simulink library "vmc"  (R2021b)
settings: Solver=VariableStepAuto  StartTime=0.0  StopTime=10.0  RelTol=1e-3
undefined symbols (not defined in the file or in its folder): AVMC_ACCDeltaTqIGain_X_kph, AVMC_ACCDeltaTqIGain_Y_mps2, AVMC_ACCDeltaTqPGain_X_kph, AVMC_ACCDeltaTqPGain_Y_kph, AVMC_ACCLongSteadyCtrl_X_kph, AVMC_AggressJerkPCT4AT_X_kph, AVMC_AggressJerkPCT_X_kph, AVMC_AggressLimitPCT4AT_X_kph, AVMC_AggressLimitPCT_X_kph, AVMC_CCLongSteadyCtrl_X_kph, AVMC_DISCDeltaTqIGain_X_kph, AVMC_DISCDeltaTqIGain_Y_mps2, AVMC_DISCDeltaTqPGain_X_kph, AVMC_DISCDeltaTqPGain_Y_kph, AVMC_DISCTrunAccJerk_X_s, AVMC_DISCTrunAccLimit_X_s, AVMC_ESCRegenOut_X_kph, AVMC_ESCRegenOut_Y_Deg, AVMC_ESCRegenOutEnSpd_X_Deg, AVMC_ISOAccLimit_X_mps, AVMC_ISODecLimit_X_mps, AVMC_ISOJerk_X_mps, AVMC_LatESCRegenOut_X_kph, AVMC_LatESCRegenOut_Y_Deg, AVMC_LongAccDeadZone_X_kph, AVMC_LongAccFiltTsforP2_X_Gps, AVMC_MCPresBaseTq_X_bar, AVMC_MSALongSteadyCtrl_X_kph, AVMC_MSAPedalOvrd2_X_kph, AVMC_MSAPedalOvrd_X_kph, AVMC_MSASpdBand_X_kph, AVMC_MSATqDownEndTq_X_kph, AVMC_MSATqDownTime_X_kph, AVMC_OPDDisSlideRate_X_Deg, AVMC_RDCDetectTime_X_kph, AVMC_RDCDetectTime_Y_pct, AVMC_RDCEnSlideRate_X_Deg, AVMC_RearWhlTqRatio_X_Nm, AVMC_RearWhlTqRatio_Y_gps, AVMC_RearWhlTqSlipGain_X_rat, AVMC_RearWhlTqSlipGain_Y_kph, AVMC_RearWhlTqSTRGGain_X_deg, AVMC_RearWhlTqSTRGGain_Y_kph, AVMC_RWSRrTSA2RWSPos_X_deg, AVMC_RWSSAS2FrtTSA_X_deg, AVMC_RWSVehSPD2RWSCoef_X_kph, AVMC_SoftJerkPCT_X_kph, AVMC_SoftLimitPCT_X_kph, AVMC_StESCYaw_X_kph, AVMC_StESCYaw_Y_Deg, AVMC_StESCYawCom_X_kph, AVMC_StESCYawCom_Y_Gps, AVMC_TMSpdBaseTq_X_rpm, AVMC_VehHoldBDecMap_X_kph, AVMC_VehHoldDecCtrlTime_X_kph, AVMC_VehHoldMCPPass_X_deg, C_TASK_10MS_S, C_TASK_5MS_S, DEG2RAD, ENUM_ACCAVAIL_AVAILABLE ... (+409)
libraries: hcu_lib x74, simulink x68, simulink_extras x3, $bdroot x2
(part 8 of 15)

== system vmc/VMC/VMC/CruiseControlFunction/CCDemandTorqueCalculation ==
  VVMC_FeatSetSpdForCalcu_kph : Inport
  VINP_VehSpeed_kph : Inport  Port=2
  VVMC_CruzActive_flg : Inport  Port=3
  VTQD_DriverWhlTqDem_Nm : Inport  Port=4
  VVMC_LongAcc_Gps : Inport  Port=5
  VVMC_CCPedalOvrd_flg : Inport  Port=6
  VVMC_CalMeterSpeed_kph : Inport  Port=7
  VVMC_FeatArbitrFinal_enum : Inport  Port=8
  VVMC_ActACCRequiredAccel_mps2 : Inport  Port=9
  VVMC_MeterIndSpeedForCalcu_kph : Inport  Port=10
  VVMC_SafetyCtrl_flg : Inport  Port=11
  VTQR_FrTMTqReq_Nm : Inport  Port=12
  VTQR_RrTMTqReq_Nm : Inport  Port=13
  VVMC_TotalAvailBrkRgnTq_Nm : Inport  Port=14
  AND12 : Logic  AllPortsSameDT=off  OutDataTypeStr=boolean
  Abs3 : Abs
  Abs4 : Abs
  Add{8,12,16,20..21} (5 alike) : Sum
  Add22 : Sum  Inputs=+-
  Add23 : Sum  Inputs=+-
  Cast To Single4 : DataTypeConversion  OutDataTypeStr=single
  Cast To Single5 : DataTypeConversion  OutDataTypeStr=single
  Constant1 : Constant  Value=KVMC_CCTqUpLim_Nm
  Constant104 : Constant  Value=ZERO_FLOAT
  Constant105 : Constant  Value=KTQD_RrTMTotalGearRatio_gain
  Constant106 : Constant  Value=KTQR_RrTMGearEff_c
  Constant107 : Constant  Value=KVMC_GravityValue_mps2
  Constant2 : Constant  Value=KVMC_CCTqLowLim_Nm
  Constant3 : Constant  Value=ZERO_FLOAT
  Constant36 : Constant  Value=KVMC_AccDevLowLim_mps2
  Constant38 : Constant  Value=KVMC_AccDevUpLim_mps2
  Constant4 : Constant  Value=KVMC_CCDISCPGainSW_flg
  Constant40 : Constant  Value=KVMC_CCSpdDevUpLim_kph
  Constant5 : Constant  Value=KVMC_CCTqUpLim_Nm
  Constant56 : Constant  Value=KVMC_CCSpdDevLowLim_kph
  Constant58 : Constant  Value=KVMC_Veh2MeterSpdFactor_enum
  Constant59 : Constant  Value=KVMC_Veh2MeterSpdOffset_enum
  Constant6 : Constant  Value=KVMC_CCTqLowLim_Nm
  Constant64 : Constant  Value=KVMC_TqSafetyCtrl_flg
  Constant65 : Constant  Value=KVMC_Veh2MeterSpdLoFactor_enum
  Constant7 : Constant  Value=ZERO_FLOAT
  Constant71 : Constant  Value=KTQR_FrTMGearEff_c
  Constant76 : Constant  Value=KTQD_FrTMTotalGearRatio_gain
  Data Type Conversion1 : DataTypeConversion  OutDataTypeStr=single
  Detect Decrease3 : simulink/Logic and Bit Operations/Detect Decrease  vinit=0.0  OutDataTypeStr=boolean
  Detect Increase3 : simulink/Logic and Bit Operations/Detect Increase  vinit=0.0  OutDataTypeStr=boolean
  Divide11 : Product  Inputs=**
  Divide12 : Product  Inputs=**
  Divide4 : Product  Inputs=***
  Divide7 : Product  Inputs=***
  InitialCondition: 1 : UnitDelay  SampleTime=-1  HasFrameUpgradeWarning=on
  Logical Operator1 : Logic  Operator=OR  AllPortsSameDT=off  OutDataTypeStr=boolean
  MVMC_DISCDeltaTqIGain_Z_Nm : Lookup_n-D  BreakpointsForDimension1=AVMC_DISCDeltaTqIGain_Y_mps2  BreakpointsForDimension2=AVMC_DISCDeltaTqIGain_X_kph  Table=MVMC_DISCDeltaTqIGain_Z_Nm  InternalRulePriority=Speed  RndMeth=Simplest  InputSameDT=on
      settings: InputPortMap=u0,u1
  MVMC_DISCDeltaTqPGain_Z_Nm : Lookup_n-D  BreakpointsForDimension1=AVMC_DISCDeltaTqPGain_Y_kph  BreakpointsForDimension2=AVMC_DISCDeltaTqPGain_X_kph  BreakpointsForDimension3=[5, 7]  Table=MVMC_DISCDeltaTqPGain_Z_Nm  ExtrapMethod=Clip  InternalRulePriority=Speed  RndMeth=Simplest  InputSameDT=on
      settings: InputPortMap=u0,u1
  Max : MinMax  Function=max  Inputs=2
  Max1 : MinMax  Function=max  Inputs=2
  Product2 : Product
  Relational Operator18 : RelationalOperator  Operator=<=  OutDataTypeStr=boolean  RndMeth=Simplest
  Saturation Dynamic{1,7..9} (4 alike) : simulink/Discontinuities/Saturation Dynamic  OutMin=[]  OutMax=[]  OutDataTypeStr=Inherit: Same as second input  OutDataType=fixdt(1, 16)  OutScaling=2^-10  DoSatur=off
  Switch{,2,5,7} (4 alike) : Switch  Criteria=u2 > Threshold
  Switch1 : Switch  Criteria=u2 > Threshold  Threshold=KVMC_Veh2MeterSpdLoBdy_kph
  Unit Delay3 : UnitDelay  SampleTime=-1  HasFrameUpgradeWarning=on
  u2 > 0 (3)1 : Switch  Criteria=u2 > Threshold
  u2 > 0 (4)1 : Switch  Criteria=u2 > Threshold
  VVMC_CruzWhlTqCal_Nm : Outport
  wires:
  VVMC_FeatSetSpdForCalcu_kph/1 -> [VVMC_FeatSetSpdForCalcu_kph]
  VTQD_DriverWhlTqDem_Nm/1 -> [VTQD_DriverWhlTqDem_Nm]
  VVMC_CruzActive_flg/1 -> [VVMC_CruzActive_flg]
  VINP_VehSpeed_kph/1 -> [VINP_VehSpeed_kph]
  [VVMC_CruzWhlTqCal_Nm] -> VVMC_CruzWhlTqCal_Nm/1
  VVMC_LongAcc_Gps/1 -> [VVMC_LongAcc_Gps]
  VVMC_CCPedalOvrd_flg/1 -> [VVMC_CCPedalOvrd_flg]
  VVMC_CalMeterSpeed_kph/1 -> [VVMC_CalMeterSpeed_kph]
  VVMC_FeatArbitrFinal_enum/1 -> [VVMC_FeatArbitrFinal_enum]
  VVMC_ActACCRequiredAccel_mps2/1 -> [VVMC_CCReqAcc_mps2]
  VVMC_MeterIndSpeedForCalcu_kph/1 -> [VVMC_MeterIndSpeedForCalcu_kph]
  VVMC_SafetyCtrl_flg/1 -> [VVMC_SafetyCtrl_flg]
  Switch5/1 -> Cast To Single5/1
  Detect Decrease3/1 -> Logical Operator1/2
  Divide4/1 -> Add16/1
  [VVMC_CruzActive_flg] -> Detect Increase3/1
  [VVMC_FeatSetSpdForCalcu_kph] -> MVMC_DISCDeltaTqPGain_Z_Nm/2
  Data Type Conversion1/1 -> Add23/1
  u2 > 0 (3)1/1 -> Switch5/1
  Constant71/1 -> Divide4/3
  Constant106/1 -> Divide7/3
  [VVMC_SafetyCtrl_flg] -> AND12/2
  Saturation Dynamic9/1 -> MVMC_DISCDeltaTqPGain_Z_Nm/1
  Relational Operator18/1 -> u2 > 0 (4)1/2
  [VVMC_LastCCWhlTqCalW_Nm] -> Abs3/1, u2 > 0 (4)1/1
  u2 > 0 (4)1/1 -> u2 > 0 (3)1/1
  [VTQR_RrTMTqReq_Nm] -> Divide7/1
  [VVMC_LastCCWhlTqCalW_Nm] -> Add12/1
  MVMC_DISCDeltaTqIGain_Z_Nm/1 -> [VVMC_CCIGainDeltaTq_Nm]
  Add23/1 -> Saturation Dynamic9/2
  Constant104/1 -> Switch5/3
  InitialCondition: 1/1 -> [VVMC_LastCCWhlTqCalW_Nm]  "VVMC_LastCruzWhlTqCal_Nm"
  Detect Increase3/1 -> Logical Operator1/1
  [VINP_VehSpeed_kph] -> MVMC_DISCDeltaTqIGain_Z_Nm/2
  [VVMC_CCIGainDeltaTq_Nm] -> Add12/2
  Abs4/1 -> Relational Operator18/2
  Saturation Dynamic7/1 -> InitialCondition: 1/1, Add21/2
  Abs3/1 -> Relational Operator18/1
  [VTQR_FrTMTqReq_Nm] -> Divide4/1
  Saturation Dynamic8/1 -> MVMC_DISCDeltaTqIGain_Z_Nm/1
  [VVMC_CCIGainDeltaTq_Nm] -> Add20/2
  Constant76/1 -> Divide4/2
  Divide7/1 -> Add16/2
  AND12/1 -> u2 > 0 (3)1/2
  Add20/1 -> Switch7/1
  Constant105/1 -> Divide7/2
  [VVMC_CruzActive_flg] -> Switch5/2
  [VVMC_CCPedalOvrd_flg] -> Unit Delay3/1
  Cast To Single5/1 -> Saturation Dynamic7/2
  Switch7/1 -> Cast To Single4/1
  Add12/1 -> Switch7/3
  Constant40/1 -> Saturation Dynamic9/1
  Constant5/1 -> Saturation Dynamic7/1
  Add16/1 -> Add20/1
  Unit Delay3/1 -> Detect Decrease3/1
  [VVMC_CCReqAcc_mps2] -> Add22/1
  Add22/1 -> Saturation Dynamic8/2
  Constant107/1 -> Product2/2
  Constant64/1 -> AND12/1
  [VVMC_FeatSetSpdForCalcu_kph] -> Data Type Conversion1/1
  Logical Operator1/1 -> Switch7/2
  Constant38/1 -> Saturation Dynamic8/1
  Product2/1 -> Add22/2
  [VVMC_LongAcc_Gps] -> Product2/1
  Constant36/1 -> Saturation Dynamic8/3
  Constant6/1 -> Max/1
  Constant56/1 -> Saturation Dynamic9/3
  Cast To Single4/1 -> u2 > 0 (4)1/3, Abs4/1, u2 > 0 (3)1/3
  VTQR_FrTMTqReq_Nm/1 -> [VTQR_FrTMTqReq_Nm]
  VTQR_RrTMTqReq_Nm/1 -> [VTQR_RrTMTqReq_Nm]
  VVMC_TotalAvailBrkRgnTq_Nm/1 -> [VVMC_TotalAvailBrkRgnTq_Nm]
  [VVMC_TotalAvailBrkRgnTq_Nm] -> Max/2
  Max/1 -> Saturation Dynamic7/3
  Switch/1 -> [VVMC_CCPGainDeltaTq_Nm]
  Switch2/1 -> Add21/1
  [VVMC_CCPGainDeltaTq_Nm] -> Switch2/1
  Constant4/1 -> Switch2/2
  Constant7/1 -> Switch2/3
  Saturation Dynamic1/1 -> [VVMC_CruzWhlTqCal_Nm]  "VVMC_CruzWhlTqCal_Nm"
  [VINP_VehSpeed_kph] -> Divide11/2, Switch1/2, Divide12/1
  Switch1/1 -> Add23/2
  Constant59/1 -> Add8/1
  Add8/1 -> Switch1/1
  Constant58/1 -> Divide11/1
  Constant65/1 -> Divide12/2
  Divide11/1 -> Add8/2
  Divide12/1 -> Switch1/3
  Max1/1 -> Saturation Dynamic1/3
  [VVMC_TotalAvailBrkRgnTq_Nm] -> Max1/2
  Constant2/1 -> Max1/1
  Constant1/1 -> Saturation Dynamic1/1
  Add21/1 -> Saturation Dynamic1/2
  [VVMC_CruzActive_flg] -> Switch/2
  MVMC_DISCDeltaTqPGain_Z_Nm/1 -> Switch/1
  Constant3/1 -> Switch/3

== system vmc/VMC/VMC/CruiseControlFunction/CCTorqueSourceDetermination ==
  VTQD_DriverWhlTqDem_Nm : Inport
  VVMC_CruzWhlTqCal_Nm : Inport  Port=2
  VTQD_LowIdleAccPedal_flg : Inport  Port=3
  VTQD_RegenMode_enum : Inport  Port=4
  VVMC_FeatArbitrFinal_enum : Inport  Port=5
  task_time_s : Inport  Port=6
  AND1 : Logic  Inputs=3  AllPortsSameDT=off  OutDataTypeStr=boolean
  Add : Sum
  Constant20 : Constant  Value=FALSE
  Constant21 : Constant  Value=ENUM_FEATARBITRSTA_CC
  Constant22 : Constant  Value=TRUE
  Constant23 : Constant  Value=KVMC_ACCPedalOvrdRestTime_s
  DelayEnable : hcu_lib/Basic_Blocks/DelayEnable
  Direct Lookup Table (n-D)1 : LookupNDDirect  NumberOfTableDimensions=1  Table=MVMC_ACCPedalOvrdTqHys_Y_Nm
  NOT2 : Logic  Operator=NOT  AllPortsSameDT=off  OutDataTypeStr=boolean
  OR1 : Logic  Operator=OR  AllPortsSameDT=off  OutDataTypeStr=boolean
  Relational Operator6 : RelationalOperator  Operator===  OutDataTypeStr=boolean  RndMeth=Simplest
  Relational Operator7 : RelationalOperator  Operator=>  OutDataTypeStr=boolean  RndMeth=Simplest
  Relational Operator8 : RelationalOperator  Operator=<=  OutDataTypeStr=boolean  RndMeth=Simplest
  SR_Latch : hcu_lib/Basic_Blocks/SR_Latch
  u2 > 0 (1) : Switch  Criteria=u2 > Threshold
  u2 > 0 (2) : Switch  Criteria=u2 > Threshold
  VVMC_CruzWhlTqReq_Nm : Outport
  VVMC_CCPedalOvrd_flg : Outport  Port=2
  wires:
  VTQD_DriverWhlTqDem_Nm/1 -> [VTQD_DriverWhlTqDem_Nm]
  VVMC_CruzWhlTqCal_Nm/1 -> [VVMC_CruzWhlTqCal_Nm]
  [VVMC_CruzWhlTqReq_Nm] -> VVMC_CruzWhlTqReq_Nm/1
  VTQD_LowIdleAccPedal_flg/1 -> [VTQD_LowIdleAccPedal_flg]
  [VVMC_CCPedalOvrd_flg] -> VVMC_CCPedalOvrd_flg/1
  [task_time_s] -> DelayEnable/3
  [VTQD_LowIdleAccPedal_flg] -> NOT2/1
  [VTQD_DriverWhlTqDem_Nm] -> u2 > 0 (1)/1
  [VVMC_CruzWhlTqCal_Nm] -> u2 > 0 (1)/3
  [VVMC_CruzWhlTqCal_Nm] -> Relational Operator8/2
  [VVMC_CruzWhlTqCal_Nm] -> Add/1
  u2 > 0 (2)/1 -> [VVMC_CCPedalOvrd_flg]
  Add/1 -> Relational Operator7/2
  [VTQD_DriverWhlTqDem_Nm] -> Relational Operator7/1
  [VVMC_FeatArbitrFinal_enum] -> Relational Operator6/1
  OR1/1 -> SR_Latch/2
  Relational Operator8/1 -> DelayEnable/1
  Constant23/1 -> DelayEnable/2
  u2 > 0 (1)/1 -> [VVMC_CruzWhlTqReq_Nm]
  Relational Operator7/1 -> SR_Latch/1
  [VVMC_CCPedalTqEnOvrd_flg] -> AND1/3
  NOT2/1 -> AND1/2
  Constant20/1 -> u2 > 0 (2)/3
  Relational Operator6/1 -> AND1/1
  [VTQD_RegenMode_enum] -> Direct Lookup Table (n-D)1/1
  [VTQD_DriverWhlTqDem_Nm] -> Relational Operator8/1
  DelayEnable/1 -> OR1/1
  SR_Latch/1 -> [VVMC_CCPedalTqEnOvrd_flg]
  [VTQD_LowIdleAccPedal_flg] -> OR1/2
  AND1/1 -> u2 > 0 (1)/2, u2 > 0 (2)/2
  Constant21/1 -> Relational Operator6/2
  Direct Lookup Table (n-D)1/1 -> Add/2
  Constant22/1 -> u2 > 0 (2)/1
  VTQD_RegenMode_enum/1 -> [VTQD_RegenMode_enum]
  VVMC_FeatArbitrFinal_enum/1 -> [VVMC_FeatArbitrFinal_enum]
  task_time_s/1 -> [task_time_s]

== system vmc/VMC/VMC/IMU/IMU memorized offset result ==
  VINP_MemOffsetGyroX_raw16 : Inport
  VINP_MemOffsetGyroY_raw16 : Inport  Port=2
  VINP_MemOffsetGyroZ_raw16 : Inport  Port=3
  VINP_MemOffsetAccX_raw16 : Inport  Port=4
  VINP_MemOffsetAccY_raw16 : Inport  Port=5
  VINP_MemOffsetAccZ_raw16 : Inport  Port=6
  ACCEL_FS_SEL = 001 SENSITIVITY = 2000 LSB/g : Constant  Value=2000
  Constant6 : Constant  Value=ONE_FLOAT  OutDataTypeStr=single
  Data Type Conversion : DataTypeConversion  OutDataTypeStr=uint16
  Data Type Conversion{1..6} (6 alike) : DataTypeConversion  OutDataTypeStr=single
  Data Type Conversion7 : DataTypeConversion  OutDataTypeStr=uint16
  Divide{,1..5} (6 alike) : Product  Inputs=**
  GYRO_FS_SEL = 0001 SENSITIVITY = 50 LSB/dps : Constant  Value=50
  Math Function{,1..5} (6 alike) : Math  Operator=reciprocal  SaturateOnIntegerOverflow=on
  Plus : Sum  Inputs=+-
  VVMC_MemOffsetGyroX_Dps : Outport
  VVMC_MemOffsetGyroY_Dps : Outport  Port=2
  VVMC_MemOffsetGyroZ_Dps : Outport  Port=3
  VVMC_MemOffsetAccX_G : Outport  Port=4
  VVMC_MemOffsetAccY_G : Outport  Port=5
  VVMC_MemOffsetAccZ_G : Outport  Port=6
  wires:
  VINP_MemOffsetGyroX_raw16/1 -> [VINP_MemOffsetGyroX_raw16]
  VINP_MemOffsetGyroY_raw16/1 -> [VINP_MemOffsetGyroY_raw16]
  [VINP_MemOffsetGyroX_raw16] -> Divide/1
  [VVMC_GyroFSCalSet_enum] -> Data Type Conversion1/1
  GYRO_FS_SEL = 0001 SENSITIVITY = 50 LSB/dps/1 -> Data Type Conversion/1
  Data Type Conversion/1 -> [VVMC_GyroFSCalSet_enum]  "VVMC_GyroFSCalSet_enum"
  [VVMC_GyroFSCalSet_enum] -> Data Type Conversion2/1
  [VINP_MemOffsetGyroY_raw16] -> Divide1/1
  [VINP_MemOffsetGyroZ_raw16] -> Divide2/1
  [VVMC_GyroFSCalSet_enum] -> Data Type Conversion3/1
  [VVMC_AccFSCalSet_enum] -> Data Type Conversion4/1
  [VINP_MemOffsetAccX_raw16] -> Divide3/1
  [VINP_MemOffsetAccY_raw16] -> Divide4/1
  [VVMC_AccFSCalSet_enum] -> Data Type Conversion5/1
  [VVMC_AccFSCalSet_enum] -> Data Type Conversion6/1
  [VINP_MemOffsetAccZ_raw16] -> Divide5/1
  Data Type Conversion7/1 -> [VVMC_AccFSCalSet_enum]  "VVMC_AccFSCalSet_enum"
  ACCEL_FS_SEL = 001 SENSITIVITY = 2000 LSB/g/1 -> Data Type Conversion7/1
  Divide/1 -> [VVMC_MemOffsetGyroX_Dps]  "VVMC_MemOffsetGyroX_Dps"
  Divide1/1 -> [VVMC_MemOffsetGyroY_Dps]  "VVMC_MemOffsetGyroY_Dps"
  Divide2/1 -> [VVMC_MemOffsetGyroZ_Dps]  "VVMC_MemOffsetGyroZ_Dps"
  Divide3/1 -> [VVMC_MemOffsetAccX_G]  "VVMC_MemOffsetAccX_G"
  Plus/1 -> [VVMC_MemOffsetAccZ_G]  "VVMC_MemOffsetAccZ_G"
  Divide5/1 -> Plus/1
  Constant6/1 -> Plus/2
  [VVMC_MemOffsetGyroX_Dps] -> VVMC_MemOffsetGyroX_Dps/1
  [VVMC_MemOffsetGyroY_Dps] -> VVMC_MemOffsetGyroY_Dps/1
  [VVMC_MemOffsetGyroZ_Dps] -> VVMC_MemOffsetGyroZ_Dps/1
  [VVMC_MemOffsetAccX_G] -> VVMC_MemOffsetAccX_G/1
  [VVMC_MemOffsetAccY_G] -> VVMC_MemOffsetAccY_G/1
  [VVMC_MemOffsetAccZ_G] -> VVMC_MemOffsetAccZ_G/1
  Divide4/1 -> [VVMC_MemOffsetAccY_G]  "VVMC_MemOffsetAccY_G"
  VINP_MemOffsetGyroZ_raw16/1 -> [VINP_MemOffsetGyroZ_raw16]
  VINP_MemOffsetAccX_raw16/1 -> [VINP_MemOffsetAccX_raw16]
  VINP_MemOffsetAccY_raw16/1 -> [VINP_MemOffsetAccY_raw16]
  VINP_MemOffsetAccZ_raw16/1 -> [VINP_MemOffsetAccZ_raw16]
  Math Function/1 -> Divide/2
  Math Function1/1 -> Divide1/2
  Math Function2/1 -> Divide2/2
  Math Function3/1 -> Divide3/2
  Math Function4/1 -> Divide4/2
  Math Function5/1 -> Divide5/2
  Data Type Conversion1/1 -> Math Function/1
  Data Type Conversion2/1 -> Math Function1/1
  Data Type Conversion3/1 -> Math Function2/1
  Data Type Conversion4/1 -> Math Function3/1
  Data Type Conversion5/1 -> Math Function4/1
  Data Type Conversion6/1 -> Math Function5/1

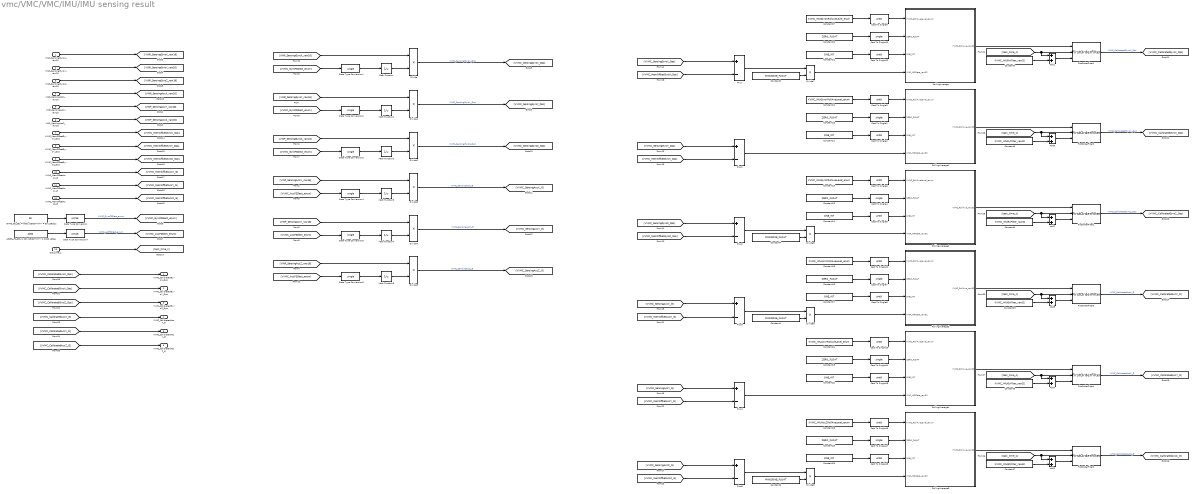
== system vmc/VMC/VMC/IMU/IMU sensing result  ==
  VINP_SensingGyroX_raw16 : Inport
  VINP_SensingGyroY_raw16 : Inport  Port=2
  VINP_SensingGyroZ_raw16 : Inport  Port=3
  VINP_SensingAccX_raw16 : Inport  Port=4
  VINP_SensingAccY_raw16 : Inport  Port=5
  VINP_SensingAccZ_raw16 : Inport  Port=6
  VVMC_MemOffsetGyroX_Dps : Inport  Port=7
  VVMC_MemOffsetGyroY_Dps : Inport  Port=8
  VVMC_MemOffsetGyroZ_Dps : Inport  Port=9
  VVMC_MemOffsetAccX_G : Inport  Port=10
  VVMC_MemOffsetAccY_G : Inport  Port=11
  VVMC_MemOffsetAccZ_G : Inport  Port=12
  task_time_s : Inport  Port=13
  ACCEL_FS_SEL = 001 SENSITIVITY = 2000 LSB/g : Constant  Value=2000
  Add{1..5,8} (6 alike) : Sum
  Cast To Single{1,4,7,10,14,17} (6 alike) : DataTypeConversion  OutDataTypeStr=single
  Cast To Single{2..3,5..6,8..9,11..13,15..16,18} (12 alike) : DataTypeConversion  OutDataTypeStr=uint8
  Constant{1..2,4,6} (4 alike) : Constant  Value=MINUSONE_FLOAT
  Constant{10,13,16,19..20,25} (6 alike) : Constant  Value=ZERO_FLOAT
  Constant{11,14,17,21..22,26} (6 alike) : Constant  Value=ONE_INT
  Constant12 : Constant  Value=KVMC_IMUGyroYRollAveLevel_enum
  Constant15 : Constant  Value=KVMC_IMUGyroZRollAveLevel_enum
  Constant18 : Constant  Value=KVMC_IMUAccXRollAveLevel_enum
  Constant23 : Constant  Value=KVMC_IMUGxFilter_raw32
  Constant24 : Constant  Value=KVMC_IMUAccYRollAveLevel_enum
  Constant27 : Constant  Value=KVMC_IMUGyroXRollAveLevel_enum
  Constant28 : Constant  Value=KVMC_IMUAccZRollAveLevel_enum
  Constant3 : Constant  Value=KVMC_IMURxFilter_raw32
  Constant5 : Constant  Value=KVMC_IMURzFilter_raw32
  Constant7 : Constant  Value=KVMC_IMUGzFilter_raw32
  Constant8 : Constant  Value=KVMC_IMUGyFilter_raw32
  Constant9 : Constant  Value=KVMC_IMURyFilter_raw32
  Data Type Conversion : DataTypeConversion  OutDataTypeStr=uint16
  Data Type Conversion{1..6} (6 alike) : DataTypeConversion  OutDataTypeStr=single
  Data Type Conversion7 : DataTypeConversion  OutDataTypeStr=uint16
  Divide{,1..9} (10 alike) : Product  Inputs=**
  FirstOrderFilter{1..6} (6 alike) : hcu_lib/Basic_Blocks/FirstOrderFilter
  GYRO_FS_SEL = 0001 SENSITIVITY = 50 LSB/dps : Constant  Value=50
  Math Function{,1..5} (6 alike) : Math  Operator=reciprocal  SaturateOnIntegerOverflow=on
  Plus{,1..5} (6 alike) : Sum  Inputs=+-
  RollingAverage : Stateflow chart  TreatAsAtomicUnit=on
  RollingAverage1 : Stateflow chart  TreatAsAtomicUnit=on
  RollingAverage2 : Stateflow chart  TreatAsAtomicUnit=on
  RollingAverage3 : Stateflow chart  TreatAsAtomicUnit=on
  RollingAverage4 : Stateflow chart  TreatAsAtomicUnit=on
  RollingAverage5 : Stateflow chart  TreatAsAtomicUnit=on
  VVMC_CalibratedGyroX_Dps : Outport
  VVMC_CalibratedGyroY_Dps : Outport  Port=2
  VVMC_CalibratedGyroZ_Dps : Outport  Port=3
  VVMC_CalibratedAccX_G : Outport  Port=4
  VVMC_CalibratedAccY_G : Outport  Port=5
  VVMC_CalibratedAccZ_G : Outport  Port=6
  wires:
  Divide4/1 -> [VVMC_SensingAccY_G]  "VVMC_SensingAccY_G"
  Divide3/1 -> [VVMC_SensingAccX_G]  "VVMC_SensingAccX_G"
  Divide2/1 -> [VVMC_SensingGyroZ_Dps]  "VVMC_SensingGyroZ_Dps"
  Divide1/1 -> [VVMC_SensingGyroY_Dps]  "VVMC_SensingGyroY_Dps"
  ACCEL_FS_SEL = 001 SENSITIVITY = 2000 LSB/g/1 -> Data Type Conversion7/1
  Data Type Conversion7/1 -> [VVMC_AccFSSlect_enum]  "VVMC_AccFSSlect_enum"
  [VINP_SensingAccZ_raw16] -> Divide5/1
  [VVMC_AccFSSlect_enum] -> Data Type Conversion5/1
  [VINP_SensingAccY_raw16] -> Divide4/1
  [VINP_SensingAccX_raw16] -> Divide3/1
  [VVMC_GyroFSSlect_enum] -> Data Type Conversion3/1
  [VINP_SensingGyroZ_raw16] -> Divide2/1
  [VINP_SensingGyroY_raw16] -> Divide1/1
  [VVMC_GyroFSSlect_enum] -> Data Type Conversion2/1
  Data Type Conversion/1 -> [VVMC_GyroFSSlect_enum]  "VVMC_GyroFSSlect_enum"
  GYRO_FS_SEL = 0001 SENSITIVITY = 50 LSB/dps/1 -> Data Type Conversion/1
  [VVMC_GyroFSSlect_enum] -> Data Type Conversion1/1
  [VINP_SensingGyroX_raw16] -> Divide/1
  VVMC_MemOffsetGyroY_Dps/1 -> [VVMC_MemOffsetGyroY_Dps]
  VVMC_MemOffsetGyroX_Dps/1 -> [VVMC_MemOffsetGyroX_Dps]
  VVMC_MemOffsetAccY_G/1 -> [VVMC_MemOffsetAccY_G]
  VVMC_MemOffsetAccZ_G/1 -> [VVMC_MemOffsetAccZ_G]
  VVMC_MemOffsetGyroZ_Dps/1 -> [VVMC_MemOffsetGyroZ_Dps]
  VVMC_MemOffsetAccX_G/1 -> [VVMC_MemOffsetAccX_G]
  VINP_SensingGyroX_raw16/1 -> [VINP_SensingGyroX_raw16]
  VINP_SensingGyroY_raw16/1 -> [VINP_SensingGyroY_raw16]
  VINP_SensingGyroZ_raw16/1 -> [VINP_SensingGyroZ_raw16]
  VINP_SensingAccX_raw16/1 -> [VINP_SensingAccX_raw16]
  VINP_SensingAccY_raw16/1 -> [VINP_SensingAccY_raw16]
  VINP_SensingAccZ_raw16/1 -> [VINP_SensingAccZ_raw16]
  Divide5/1 -> [VVMC_SensingAccZ_G]  "VVMC_SensingAccZ_G"
  Divide/1 -> [VVMC_SensingGyroX_Dps]  "VVMC_SensingGyroX_Dps"
  [VVMC_SensingGyroX_Dps] -> Plus/1
  [VVMC_MemOffsetGyroX_Dps] -> Plus/2
  [VVMC_SensingGyroY_Dps] -> Plus1/1
  [VVMC_MemOffsetGyroY_Dps] -> Plus1/2
  [VVMC_SensingGyroZ_Dps] -> Plus2/1
  [VVMC_MemOffsetGyroZ_Dps] -> Plus2/2
  [VVMC_SensingAccX_G] -> Plus3/1
  [VVMC_MemOffsetAccX_G] -> Plus3/2
  [VVMC_SensingAccY_G] -> Plus4/1
  [VVMC_MemOffsetAccY_G] -> Plus4/2
  [VVMC_SensingAccZ_G] -> Plus5/1
  [VVMC_MemOffsetAccZ_G] -> Plus5/2
  FirstOrderFilter1/1 -> [VVMC_CalibratedGyroX_Dps]  "VVMC_CalibratedGyroX_Dps"
  FirstOrderFilter5/1 -> [VVMC_CalibratedGyroY_Dps]  "VVMC_CalibratedGyroY_Dps"
  FirstOrderFilter2/1 -> [VVMC_CalibratedGyroZ_Dps]  "VVMC_CalibratedGyroZ_Dps"
  FirstOrderFilter6/1 -> [VVMC_CalibratedAccX_G]  "VVMC_CalibratedAccX_G"
  FirstOrderFilter4/1 -> [VVMC_CalibratedAccY_G]  "VVMC_CalibratedAccY_G"
  FirstOrderFilter3/1 -> [VVMC_CalibratedAccZ_G]  "VVMC_CalibratedAccZ_G"
  Math Function/1 -> Divide/2
  Math Function1/1 -> Divide1/2
  Math Function2/1 -> Divide2/2
  Math Function3/1 -> Divide3/2
  Math Function4/1 -> Divide4/2
  Math Function5/1 -> Divide5/2
  Data Type Conversion1/1 -> Math Function/1
  Data Type Conversion2/1 -> Math Function1/1
  Data Type Conversion3/1 -> Math Function2/1
  [VVMC_AccFSSlect_enum] -> Data Type Conversion4/1
  Data Type Conversion4/1 -> Math Function3/1
  Data Type Conversion5/1 -> Math Function4/1
  [VVMC_AccFSSlect_enum] -> Data Type Conversion6/1
  Data Type Conversion6/1 -> Math Function5/1
  task_time_s/1 -> [task_time_s]
  [task_time_s] -> Add8/1, FirstOrderFilter6/2
  Plus3/1 -> Divide6/1
  Constant23/1 -> Add8/2
  Add8/1 -> FirstOrderFilter6/3
  Constant1/1 -> Divide6/2
  Divide6/1 -> RollingAverage3/4(VINP_INPData_raw32)
  Divide7/1 -> RollingAverage/4(VINP_INPData_raw32)
  Constant2/1 -> Divide7/2
  Add1/1 -> FirstOrderFilter1/3
  Constant3/1 -> Add1/2
  [task_time_s] -> FirstOrderFilter1/2, Add1/1
  Plus/1 -> Divide7/1
  [task_time_s] -> Add2/1, FirstOrderFilter2/2
  Constant5/1 -> Add2/2
  Add2/1 -> FirstOrderFilter2/3
  Constant4/1 -> Divide8/2
  Divide8/1 -> RollingAverage2/4(VINP_INPData_raw32)
  Plus2/1 -> Divide8/1
  Divide9/1 -> RollingAverage5/4(VINP_INPData_raw32)
  Constant6/1 -> Divide9/2
  Add3/1 -> FirstOrderFilter3/3
  Constant7/1 -> Add3/2
  [task_time_s] -> FirstOrderFilter3/2, Add3/1
  Plus5/1 -> Divide9/1
  Add4/1 -> FirstOrderFilter4/3
  Constant8/1 -> Add4/2
  [task_time_s] -> FirstOrderFilter4/2, Add4/1
  Plus4/1 -> RollingAverage4/4(VINP_INPData_raw32)
  [task_time_s] -> Add5/1, FirstOrderFilter5/2
  Constant9/1 -> Add5/2
  Add5/1 -> FirstOrderFilter5/3
  Plus1/1 -> RollingAverage1/4(VINP_INPData_raw32)
  Constant20/1 -> Cast To Single10/1
  Constant27/1 -> Cast To Single9/1
  Cast To Single12/1 -> RollingAverage/3(ONE_INT)
  Cast To Single9/1 -> RollingAverage/1(KVMC_RollAveLevel_enum)
  Cast To Single10/1 -> RollingAverage/2(ZERO_FLOAT)
  Constant21/1 -> Cast To Single12/1
  RollingAverage/1(VVMC_RollAve_raw32) -> FirstOrderFilter1/1
  Constant11/1 -> Cast To Single2/1
  Cast To Single1/1 -> RollingAverage1/2(ZERO_FLOAT)
  Cast To Single3/1 -> RollingAverage1/1(KVMC_RollAveLevel_enum)
  Cast To Single2/1 -> RollingAverage1/3(ONE_INT)
  Constant12/1 -> Cast To Single3/1
  Constant10/1 -> Cast To Single1/1
  RollingAverage1/1(VVMC_RollAve_raw32) -> FirstOrderFilter5/1
  Constant13/1 -> Cast To Single4/1
  Constant15/1 -> Cast To Single6/1
  Constant14/1 -> Cast To Single5/1
  Cast To Single6/1 -> RollingAverage2/1(KVMC_RollAveLevel_enum)
  Cast To Single4/1 -> RollingAverage2/2(ZERO_FLOAT)
  Cast To Single5/1 -> RollingAverage2/3(ONE_INT)
  RollingAverage2/1(VVMC_RollAve_raw32) -> FirstOrderFilter2/1
  Constant17/1 -> Cast To Single8/1
  Cast To Single7/1 -> RollingAverage3/2(ZERO_FLOAT)
  Cast To Single11/1 -> RollingAverage3/1(KVMC_RollAveLevel_enum)
  Cast To Single8/1 -> RollingAverage3/3(ONE_INT)
  Constant18/1 -> Cast To Single11/1
  Constant16/1 -> Cast To Single7/1
  RollingAverage3/1(VVMC_RollAve_raw32) -> FirstOrderFilter6/1
  Constant19/1 -> Cast To Single14/1
  Constant24/1 -> Cast To Single13/1
  Cast To Single15/1 -> RollingAverage4/3(ONE_INT)
  Cast To Single13/1 -> RollingAverage4/1(KVMC_RollAveLevel_enum)
  Cast To Single14/1 -> RollingAverage4/2(ZERO_FLOAT)
  Constant22/1 -> Cast To Single15/1
  RollingAverage4/1(VVMC_RollAve_raw32) -> FirstOrderFilter4/1
  Constant26/1 -> Cast To Single18/1
  Cast To Single17/1 -> RollingAverage5/2(ZERO_FLOAT)
  Cast To Single16/1 -> RollingAverage5/1(KVMC_RollAveLevel_enum)
  Cast To Single18/1 -> RollingAverage5/3(ONE_INT)
  Constant28/1 -> Cast To Single16/1
  Constant25/1 -> Cast To Single17/1
  RollingAverage5/1(VVMC_RollAve_raw32) -> FirstOrderFilter3/1
  [VVMC_CalibratedGyroX_Dps] -> VVMC_CalibratedGyroX_Dps/1
  [VVMC_CalibratedGyroY_Dps] -> VVMC_CalibratedGyroY_Dps/1
  [VVMC_CalibratedGyroZ_Dps] -> VVMC_CalibratedGyroZ_Dps/1
  [VVMC_CalibratedAccX_G] -> VVMC_CalibratedAccX_G/1
  [VVMC_CalibratedAccY_G] -> VVMC_CalibratedAccY_G/1
  [VVMC_CalibratedAccZ_G] -> VVMC_CalibratedAccZ_G/1

== system vmc/VMC/VMC/Long Acceleration Calculation/Vehicle to Meter Speed ==
  InputSpeed : Inport
  Add4 : Sum
  Constant16 : Constant  Value=KVMC_Veh2MeterSpdFactor_enum
  Constant23 : Constant  Value=KVMC_Veh2MeterSpdOffset_enum
  Constant28 : Constant  Value=KVMC_Veh2MeterSpdLoFactor_enum
  Divide5 : Product  Inputs=**
  Divide8 : Product  Inputs=**
  Switch : Switch  Criteria=u2 > Threshold  Threshold=KVMC_Veh2MeterSpdLoBdy_kph
  OutputSpeed : Outport
  wires:
  Add4/1 -> Switch/1
  Divide5/1 -> Add4/2
  Constant16/1 -> Divide5/1
  InputSpeed/1 -> Divide5/2, Switch/2, Divide8/1
  Constant23/1 -> Add4/1
  Constant28/1 -> Divide8/2
  Divide8/1 -> Switch/3
  Switch/1 -> OutputSpeed/1

== system vmc/VMC/VMC/MSA function/Anti-Speed Limitation ==
  VINP_HoodSW_flg : Inport
  VTQD_GearActualPosn_enum : Inport  Port=2
  AND : Logic  Inputs=3  AllPortsSameDT=off  OutDataTypeStr=boolean
  Constant1 : Constant  Value=KVMC_AntiSpdLimSW_flg
  Constant2 : Constant  Value=ENUM_GEARACTUALPOSN_D
  Equal : RelationalOperator  Operator===  OutDataTypeStr=boolean  RndMeth=Simplest
  VVMC_AntiSpdLimEn_flg : Outport
  wires:
  [VINP_HoodSW_flg] -> AND/1
  Constant1/1 -> AND/3
  Equal/1 -> AND/2
  AND/1 -> [VVMC_AntiSpdLimEn_flg]  "VVMC_AntiSpdLimEn_flg"
  Constant2/1 -> Equal/2
  [VTQD_GearActualPosn_enum] -> Equal/1
  VINP_HoodSW_flg/1 -> [VINP_HoodSW_flg]
  [VVMC_AntiSpdLimEn_flg] -> VVMC_AntiSpdLimEn_flg/1
  VTQD_GearActualPosn_enum/1 -> [VTQD_GearActualPosn_enum]

== system vmc/VMC/VMC/MSA function/MSAActivationHandshake ==
  VTQD_SpdCtrlMode_enum : Inport
  VVMC_FeatArbitrFinal_enum : Inport  Port=2
  VTQD_ExternalTqAllow_flg : Inport  Port=3
  VVMC_MeterIndSpeedForCalcu_kph : Inport  Port=4
  VVMC_FeatSetSpdForCalcu_kph : Inport  Port=5
  VTQD_SWCCANCELSta_flg : Inport  Port=6
  VTQD_SWCResUpSta_flg : Inport  Port=7
  VTQD_SWCSetdownSta_flg : Inport  Port=8
  VVMC_MSAOvrdAllow_flg : Inport  Port=9
  VINP_Distanceunit_flg : Inport  Port=10
  " 1" : Constant  Value=KTQD_MSAActiveMetSpdLoMPH_mph
  " 80" : Constant  Value=KTQD_MSAActiveMetSpdLo_kph
  160 : Constant  Value=KTQD_MSAActiveMetSpdHi_kph
  2 : Constant  Value=KTQD_MSAActiveMetSpdHiMPH_mph
  AND : Logic  AllPortsSameDT=off  OutDataTypeStr=boolean
  AND1 : Logic  Operator=OR  AllPortsSameDT=off  OutDataTypeStr=boolean
  Cast To Boolean : DataTypeConversion  OutDataTypeStr=boolean
  Cast To Single : DataTypeConversion  OutDataTypeStr=uint8
  Cast To Single1 : DataTypeConversion  OutDataTypeStr=boolean
  Cast To Single2 : DataTypeConversion  OutDataTypeStr=single
  Cast To Single3 : DataTypeConversion  OutDataTypeStr=single
  Chart : Stateflow chart  TreatAsAtomicUnit=on
  Constant2 : Constant  Value=KVMC_CCMSASpdWar_kph
  Constant3 : Constant  Value=ENUM_ADASMSASTA_UNLIMIT
  Constant5 : Constant  Value=ENUM_FEATARBITRSTA_MSA
  Constant6 : Constant  Value=TRUE
  Constant7 : Constant  Value=FALSE
  Constant8 : Constant  Value=ENUM_ADASMSASTA_ACTIVE
  Detect Decrease1 : simulink/Logic and Bit Operations/Detect Decrease  vinit=0.0  OutDataTypeStr=boolean
  Detect Decrease2 : simulink/Logic and Bit Operations/Detect Decrease  vinit=0.0  OutDataTypeStr=boolean
  Detect Decrease3 : simulink/Logic and Bit Operations/Detect Decrease  vinit=0.0  OutDataTypeStr=boolean
  Relational Operator : RelationalOperator  Operator===  OutDataTypeStr=boolean  RndMeth=Simplest
  Relational Operator1 : RelationalOperator  Operator===  OutDataTypeStr=boolean  RndMeth=Simplest
  Relational Operator2 : RelationalOperator  Operator===  OutDataTypeStr=boolean  RndMeth=Simplest
  Switch2 : Switch  Criteria=u2 > Threshold
  Switch3 : Switch  Criteria=u2 > Threshold
  u2 > 0 : Switch  Criteria=u2 > Threshold
  VVMC_MSACtrlSta_enum : Outport
  VVMC_MSASpdWar_flg : Outport  Port=2
  VVMC_MSAActive_flg : Outport  Port=3
  wires:
  AND1/1 -> AND/2
  Relational Operator2/1 -> AND1/2
  Constant3/1 -> Relational Operator2/2
  [VVMC_MSACtrlSta_enum] -> Relational Operator2/1
  [VVMC_MSAOvrdAllow_flg] -> Chart/9(VVMC_MSAOvrdAllow_flg)
  VVMC_MSAOvrdAllow_flg/1 -> [VVMC_MSAOvrdAllow_flg]
  Cast To Single/1 -> [VVMC_MSACtrlSta_enum]  "VVMC_MSACtrlSta_enum"
  Cast To Boolean/1 -> [VVMC_MSAActive_flg]  "VVMC_MSAActive_flg"
  Cast To Single1/1 -> [VVMC_MSASpdWar_flg]  "VVMC_MSASpdWar_flg"
  VVMC_MeterIndSpeedForCalcu_kph/1 -> [VVMC_MeterIndSpeedForCalcu_kph]
  VVMC_FeatSetSpdForCalcu_kph/1 -> [VVMC_FeatSetSpdForCalcu_kph]
  VTQD_SWCCANCELSta_flg/1 -> [VTQD_SWCCANCELSta_flg]
  VTQD_ExternalTqAllow_flg/1 -> [VTQD_ExternalTqAllow_flg]
  VVMC_FeatArbitrFinal_enum/1 -> [VVMC_FeatArbitrFinal_enum]
  [VVMC_MSAActive_flg] -> VVMC_MSAActive_flg/1
  [VVMC_MSASpdWar_flg] -> VVMC_MSASpdWar_flg/1
  [VVMC_MSACtrlSta_enum] -> VVMC_MSACtrlSta_enum/1
  u2 > 0/1 -> Cast To Boolean/1
  Chart/2(VVMC_MSASpdWar_flg) -> Cast To Single1/1
  Chart/1(VVMC_MSACtrlSta_enum) -> Cast To Single/1
  Detect Decrease1/1 -> Chart/8(VVMC_DetectSWCCANCEL_flg)  "VVMC_DetectSWCCANCEL_flg"
  [VTQD_SWCCANCELSta_flg] -> Detect Decrease1/1
  Constant2/1 -> Chart/7(KVMC_CCMSASpdWar_kph)
  [VVMC_FeatSetSpdForCalcu_kph] -> Chart/6(VVMC_FeatSetSpdForCalcu_kph)
  Switch3/1 -> Cast To Single3/1
  [VVMC_MeterIndSpeedForCalcu_kph] -> Chart/4(VVMC_MeterIndSpeedForCalcu_kph)
  Switch2/1 -> Cast To Single2/1
  [VTQD_ExternalTqAllow_flg] -> Chart/2(VTQD_ExternalTqAllow_flg)
  VTQD_SpdCtrlMode_enum/1 -> [VTQD_SpdCtrlMode_enum]
  [VTQD_SpdCtrlMode_enum] -> Chart/1(VTQD_SpdCtrlMode_enum)
  Constant8/1 -> Relational Operator1/2
  AND/1 -> u2 > 0/2
  [VVMC_FeatArbitrFinal_enum] -> Relational Operator/1
  Constant5/1 -> Relational Operator/2
  [VVMC_MSACtrlSta_enum] -> Relational Operator1/1
  Constant6/1 -> u2 > 0/1
  Relational Operator1/1 -> AND1/1
  Relational Operator/1 -> AND/1
  Constant7/1 -> u2 > 0/3
  [VTQD_SWCResUpSta_flg] -> Detect Decrease2/1
  Detect Decrease2/1 -> Chart/10(VVMC_DetectSWCRes_flg)  "VVMC_DetectSWCRes_flg"
  [VTQD_SWCSetdownSta_flg] -> Detect Decrease3/1
  Detect Decrease3/1 -> Chart/11(VVMC_DetectSWCSet_flg)  "VVMC_DetectSWCSet_flg"
  VTQD_SWCSetdownSta_flg/1 -> [VTQD_SWCSetdownSta_flg]
  VTQD_SWCResUpSta_flg/1 -> [VTQD_SWCResUpSta_flg]
  [VINP_Distanceunit_flg] -> Switch2/2
  2/1 -> Switch2/1
  160/1 -> Switch2/3
  " 80"/1 -> Switch3/3
  " 1"/1 -> Switch3/1
  [VINP_Distanceunit_flg] -> Switch3/2
  VINP_Distanceunit_flg/1 -> [VINP_Distanceunit_flg]
  Cast To Single2/1 -> Chart/3(KVMC_MSAActiveMetSpdHi_kph)
  Cast To Single3/1 -> Chart/5(KVMC_MSAActiveMetSpdLo_kph)

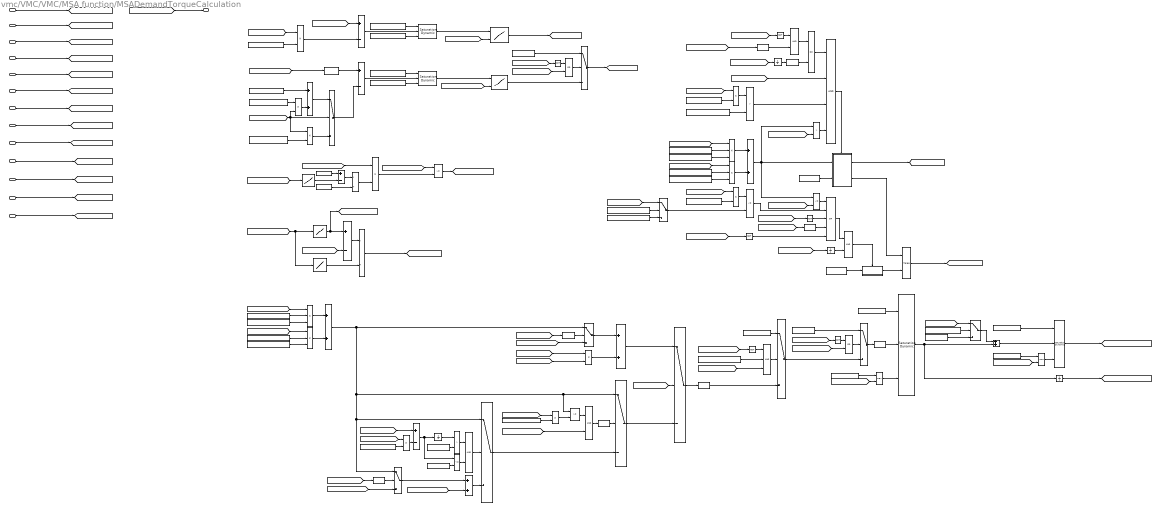
== system vmc/VMC/VMC/MSA function/MSADemandTorqueCalculation ==
  VVMC_FeatSetSpdForCalcu_kph : Inport
  VINP_VehSpeed_kph : Inport  Port=2
  VVMC_MSAActive_flg : Inport  Port=3
  VTQD_DriverWhlTqDem_Nm : Inport  Port=4
  VVMC_LongAcc_Gps : Inport  Port=5
  VVMC_MeterIndSpeedForCalcu_kph : Inport  Port=6
  VVMC_ActACCRequiredAccel_mps2 : Inport  Port=7
  VTQR_FrTMTqReq_Nm : Inport  Port=8
  VTQR_RrTMTqReq_Nm : Inport  Port=9
  VVMC_MSAPedalOvrd_flg : Inport  Port=10
  task_time_s : Inport  Port=11
  VTQD_LowIdleAccPedal_flg : Inport  Port=12
  VVMC_TotalAvailBrkRgnTq_Nm : Inport  Port=13
  1-D Lookup Table4 : Lookup_n-D  NumberOfTableDimensions=1  BreakpointsForDimension1=AVMC_MSASpdBand_X_kph  Table=MVMC_MSASpdBand_Y_pct  InternalRulePriority=Speed  RndMeth=Simplest  InputSameDT=on
  AND1 : Logic  Inputs=4  AllPortsSameDT=off  OutDataTypeStr=boolean
  AND2 : Logic  Operator=OR  Inputs=5  AllPortsSameDT=off  OutDataTypeStr=boolean
  AND{4..6,8} (4 alike) : Logic  AllPortsSameDT=off  OutDataTypeStr=boolean
  AND7 : Logic  Inputs=3  AllPortsSameDT=off  OutDataTypeStr=boolean
  Add{,6,10,22..23} (5 alike) : Sum  Inputs=+-
  Add{1..3,5,8,12} (6 alike) : Sum
  Cast To Single4 : DataTypeConversion  OutDataTypeStr=single
  Cast To Single5 : DataTypeConversion  OutDataTypeStr=single
  Constant1 : Constant  Value=KVMC_MSAEnCtrlTargetAccSW_flg
  Constant10 : Constant  Value=KVMC_MSATqUpLim_Nm  OutDataTypeStr=single
  Constant{18,20,31,107} (4 alike) : Constant  Value=KVMC_GravityValue_mps2
  Constant11 : Constant  Value=KVMC_MSATqUpLim_Nm  OutDataTypeStr=single
  Constant{6..7,12,41..42} (5 alike) : Constant  Value=ZERO_FLOAT
  Constant17 : Constant  Value=KVMC_MSAEnCtrlTargetAcc_mps2
  Constant19 : Constant  Value=KVMC_MSAEnCtrlTargetAcc_mps2
  Constant2 : Constant  Value=pct
  Constant21 : Constant  Value=TRUE
  Constant22 : Constant  Value=KTQD_RrTMTotalGearRatio_gain
  Constant23 : Constant  Value=KTQR_RrTMGearEff_c
  Constant24 : Constant  Value=KTQR_FrTMGearEff_c
  Constant25 : Constant  Value=KTQD_FrTMTotalGearRatio_gain
  Constant26 : Constant  Value=FALSE
  Constant3 : Constant  Value=pct
  Constant32 : Constant  Value=KTQD_RrTMTotalGearRatio_gain
  Constant33 : Constant  Value=KTQR_RrTMGearEff_c
  Constant34 : Constant  Value=KTQR_FrTMGearEff_c
  Constant35 : Constant  Value=KTQD_FrTMTotalGearRatio_gain
  Constant36 : Constant  Value=KVMC_AccDevLowLim_mps2
  Constant38 : Constant  Value=KVMC_AccDevUpLim_mps2
  Constant39 : Constant  Value=KVMC_MSATqLowLim_Nm  OutDataTypeStr=single
  Constant4 : Constant  Value=KVMC_MSAPGainSW_flg
  Constant40 : Constant  Value=KVMC_MSASpdDevUpLim_kph
  Constant49 : Constant  Value=KVMC_MSATqUpLim_Nm  OutDataTypeStr=single
  Constant5 : Constant  Value=KVMC_MSACreepSW2_flg
  Constant56 : Constant  Value=KVMC_MSASpdDevLowLim_kph
  Constant58 : Constant  Value=KVMC_Veh2MeterSpdFactor_enum
  Constant59 : Constant  Value=KVMC_Veh2MeterSpdOffset_enum
  Constant65 : Constant  Value=KVMC_Veh2MeterSpdLoFactor_enum
  Constant8 : Constant  Value=KVMC_MSATqLowLim_Nm  OutDataTypeStr=single
  Constant9 : Constant  Value=KVMC_MSATqDownEndTqRatio_pct
  Data Type Conversion1 : DataTypeConversion  OutDataTypeStr=single
  Detect Decrease1 : simulink/Logic and Bit Operations/Detect Decrease  vinit=0.0  OutDataTypeStr=boolean
  Detect Increase{,1..4} (5 alike) : simulink/Logic and Bit Operations/Detect Increase  vinit=0.0  OutDataTypeStr=boolean
  Divide : Product  Inputs=*/
  Divide{1..3,5} (4 alike) : Product  Inputs=***
  Divide{4,6,11..12} (4 alike) : Product  Inputs=**
  InitialCondition: 1 : UnitDelay  SampleTime=-1  HasFrameUpgradeWarning=on
  Logical Operator2 : Logic  Operator=OR  AllPortsSameDT=off  OutDataTypeStr=boolean
  MVMC_DISCDeltaTqIGain_Z_Nm : Lookup_n-D  BreakpointsForDimension1=AVMC_DISCDeltaTqIGain_Y_mps2  BreakpointsForDimension2=AVMC_DISCDeltaTqIGain_X_kph  Table=MVMC_DISCDeltaTqIGain_Z_Nm  InternalRulePriority=Speed  RndMeth=Simplest  InputSameDT=on
      settings: InputPortMap=u0,u1
  MVMC_DISCDeltaTqPGain_Z_Nm : Lookup_n-D  BreakpointsForDimension1=AVMC_DISCDeltaTqPGain_Y_kph  BreakpointsForDimension2=AVMC_DISCDeltaTqPGain_X_kph  BreakpointsForDimension3=[5, 7]  Table=MVMC_DISCDeltaTqPGain_Z_Nm  ExtrapMethod=Clip  InternalRulePriority=Speed  RndMeth=Simplest  InputSameDT=on
      settings: InputPortMap=u0,u1
  MVMC_MSATqDownEndTq_Y_Nm : Lookup_n-D  NumberOfTableDimensions=1  BreakpointsForDimension1=AVMC_MSATqDownEndTq_X_kph  Table=MVMC_MSATqDownEndTq_Y_Nm  InternalRulePriority=Speed  RndMeth=Simplest  InputSameDT=on
  MVMC_MSATqDownTime_Y_s : Lookup_n-D  NumberOfTableDimensions=1  BreakpointsForDimension1=AVMC_MSATqDownTime_X_kph  Table=MVMC_MSATqDownTime_Y_s  InternalRulePriority=Speed  RndMeth=Simplest  InputSameDT=on
  Max : MinMax  Function=max  Inputs=2
  Max1 : MinMax  Function=max  Inputs=2
  Merge : Merge
  NOT{,1..5} (6 alike) : Logic  Operator=NOT  AllPortsSameDT=off  OutDataTypeStr=boolean
  OR : Logic  Operator=OR  AllPortsSameDT=off  OutDataTypeStr=boolean
  OR1 : Logic  Operator=OR  AllPortsSameDT=off  OutDataTypeStr=boolean
  Product{2..5,13} (5 alike) : Product
  Product14 : Product  Inputs=*/
  Relational Operator : RelationalOperator  Operator=>  OutDataTypeStr=boolean  RndMeth=Simplest
  Relational Operator1 : RelationalOperator  Operator=<=  OutDataTypeStr=boolean  RndMeth=Simplest
  Relational Operator10 : RelationalOperator  OutDataTypeStr=boolean  RndMeth=Simplest
  Relational Operator2 : RelationalOperator  Operator=>  OutDataTypeStr=boolean  RndMeth=Simplest
  Relational Operator3 : RelationalOperator  Operator=<=  OutDataTypeStr=boolean  RndMeth=Simplest
  Relational Operator4 : RelationalOperator  Operator=>  OutDataTypeStr=boolean  RndMeth=Simplest
  Relational Operator5 : RelationalOperator  Operator=<=  OutDataTypeStr=boolean  RndMeth=Simplest
  Relational Operator8 : RelationalOperator  OutDataTypeStr=boolean  RndMeth=Simplest
  Saturation Dynamic{1,7..9} (4 alike) : simulink/Discontinuities/Saturation Dynamic  OutMin=[]  OutMax=[]  OutDataTypeStr=Inherit: Same as second input  OutDataType=fixdt(1, 16)  OutScaling=2^-10  DoSatur=off
  Switch{,1..6,8,10,12} (10 alike) : Switch  Criteria=u2 > Threshold
  Switch7 : Switch  Criteria=u2 > Threshold  Threshold=KVMC_Veh2MeterSpdLoBdy_kph
  Triggered Subsystem : Subsystem  TreatAsAtomicUnit=on
  Triggered Subsystem1 : Subsystem  TreatAsAtomicUnit=on
  Unit Delay : UnitDelay  SampleTime=-1  HasFrameUpgradeWarning=on
  Unit Delay2 : UnitDelay  SampleTime=-1  HasFrameUpgradeWarning=on
  Unit Delay3 : UnitDelay  SampleTime=-1  HasFrameUpgradeWarning=on
  VVMC_MSAWhlTqCal_Nm : Outport
  wires:
  [VVMC_MSAPedalOvrd_flg] -> NOT3/1
  NOT3/1 -> AND6/1
  AND6/1 -> Logical Operator2/1
  Unit Delay3/1 -> AND5/2
  [VVMC_MSATqDown_flg] -> Unit Delay3/1
  Detect Increase4/1 -> AND2/4
  NOT1/1 -> AND2/5
  [VVMC_MSAActive_flg] -> AND1/2
  AND4/1 -> Switch12/2
  Relational Operator4/1 -> AND4/1
  Relational Operator5/1 -> AND4/2
  Switch12/1 -> Switch4/3
  Constant42/1 -> Relational Operator5/2
  Constant41/1 -> Relational Operator4/2
  Unit Delay/1 -> Relational Operator4/1
  Add10/1 -> Unit Delay/1, Relational Operator5/1
  [VVMC_LongAcc_Gps] -> Product5/1
  Constant31/1 -> Product5/2
  [VVMC_MSAReqAcc_mps2] -> Add10/1
  Product5/1 -> Add10/2
  VTQD_LowIdleAccPedal_flg/1 -> [VTQD_LowIdleAccPedal_flg]
  Relational Operator3/1 -> AND2/1
  [VVMC_MSATqDownEndTq_Nm] -> Relational Operator3/2
  [VVMC_MSAPedalOvrd_flg] -> Detect Increase4/1
  Switch/1 -> Add5/1
  [VVMC_LastMSAWhlTqCalW_Nm] -> Switch/3
  Detect Increase/1 -> Switch/2
  [VVMC_MSATqDown_flg] -> Detect Increase/1
  Logical Operator2/1 -> AND1/1
  Detect Decrease1/1 -> Logical Operator2/2
  [VVMC_MSAPedalOvrd_flg] -> Unit Delay2/1
  Unit Delay2/1 -> Detect Decrease1/1
  Divide6/1 -> Add5/2
  Add5/1 -> Switch10/1
  [task_time_s] -> Divide6/2
  [VVMC_MSATqDownSlope_Nmps] -> Divide6/1
  task_time_s/1 -> [task_time_s]
  Constant33/1 -> Divide5/3
  Divide3/1 -> Add2/1
  [VTQR_RrTMTqReq_Nm] -> Divide5/1
  Constant35/1 -> Divide3/2
  Constant32/1 -> Divide5/2
  Divide5/1 -> Add2/2
  Constant34/1 -> Divide3/3
  [VTQR_FrTMTqReq_Nm] -> Divide3/1
  [VVMC_MSATqDown_flg] -> Switch10/2
  Divide/1 -> [VVMC_MSATqDownSlope_Nmps]  "VVMC_MSATqDownSlope_Nmps"
  MVMC_MSATqDownTime_Y_s/1 -> Divide/2
  Add/1 -> Divide/1
  MVMC_MSATqDownEndTq_Y_Nm/1 -> [VVMC_MSATqDownEndTq_Nm], Add/1
  [VVMC_MSATqDownEnTq_Nm] -> Add/2
  [VVMC_MSATqDownEndTq_Nm] -> Relational Operator2/2
  Relational Operator2/1 -> AND1/4
  Triggered Subsystem/1(Out1) -> [VVMC_MSATqDownEnTq_Nm]  "VVMC_MSATqDownEnTq_Nm"
  Triggered Subsystem/2(Out2) -> Merge/1
  Triggered Subsystem1/1(Out1) -> Merge/2
  Merge/1 -> [VVMC_MSATqDown_flg]  "VVMC_MSATqDown_flg"
  Relational Operator1/1 -> AND2/2
  NOT/1 -> AND2/3
  [VVMC_MSAActive_flg] -> NOT/1
  Constant26/1 -> Triggered Subsystem1/1(In1)
  AND2/1 -> AND5/1
  Add1/1 -> Triggered Subsystem/1(In1), Relational Operator3/1, Relational Operator2/1
  [VTQR_FrTMTqReq_Nm] -> Divide1/1
  Constant24/1 -> Divide1/3
  Divide2/1 -> Add1/2
  Constant22/1 -> Divide2/2
  Constant25/1 -> Divide1/2
  [VTQR_RrTMTqReq_Nm] -> Divide2/1
  Constant23/1 -> Divide2/3
  Divide1/1 -> Add1/1
  Constant21/1 -> Triggered Subsystem/2(In2)
  AND1/1 -> Triggered Subsystem/Trigger
  Constant20/1 -> Product4/2
  [VVMC_LongAcc_Gps] -> Product4/1
  Product4/1 -> Relational Operator1/1
  Switch1/1 -> Relational Operator1/2
  Relational Operator/1 -> AND1/3
  Detect Increase2/1 -> AND6/2
  [VVMC_MSAInCtrlSpd_flg] -> Detect Increase2/1
  Constant17/1 -> Relational Operator/2
  Product3/1 -> Relational Operator/1
  [VVMC_LongAcc_Gps] -> Product3/1
  Constant18/1 -> Product3/2
  VVMC_MSAPedalOvrd_flg/1 -> [VVMC_MSAPedalOvrd_flg]
  VTQR_RrTMTqReq_Nm/1 -> [VTQR_RrTMTqReq_Nm]
  VTQR_FrTMTqReq_Nm/1 -> [VTQR_FrTMTqReq_Nm]
  VVMC_ActACCRequiredAccel_mps2/1 -> [VVMC_MSAReqAcc_mps2]
  [VVMC_FeatSetSpdForCalcu_kph] -> MVMC_DISCDeltaTqPGain_Z_Nm/2
  Switch3/1 -> Cast To Single5/1
  Saturation Dynamic9/1 -> MVMC_DISCDeltaTqPGain_Z_Nm/1
  [VVMC_MSAIGainDeltaTq_Nm] -> Add12/2
  InitialCondition: 1/1 -> [VVMC_LastMSAWhlTqCalW_Nm]  "VVMC_MSAWhlTqCalDelay_Nm"
  Add23/1 -> Saturation Dynamic9/2
  Switch6/1 -> Add12/1
  Saturation Dynamic8/1 -> MVMC_DISCDeltaTqIGain_Z_Nm/1
  Constant38/1 -> Saturation Dynamic8/1
  MVMC_DISCDeltaTqIGain_Z_Nm/1 -> [VVMC_MSAIGainDeltaTq_Nm]
  Data Type Conversion1/1 -> Add23/1
  Constant40/1 -> Saturation Dynamic9/1
  Saturation Dynamic7/1 -> InitialCondition: 1/1, Add3/2
  Add12/1 -> Switch12/3
  Constant39/1 -> Max/1
  Product2/1 -> Add22/2
  [VVMC_MSAReqAcc_mps2] -> Add22/1
  Constant107/1 -> Product2/2
  Cast To Single5/1 -> Saturation Dynamic7/2
  [VVMC_FeatSetSpdForCalcu_kph] -> Data Type Conversion1/1
  Constant36/1 -> Saturation Dynamic8/3
  [VINP_VehSpeed_kph] -> MVMC_DISCDeltaTqIGain_Z_Nm/2
  [VVMC_LongAcc_Gps] -> Product2/1
  Switch8/1 -> [VVMC_MSAPGainDeltaTq_Nm]
  Constant56/1 -> Saturation Dynamic9/3
  Switch10/1 -> Cast To Single4/1
  Add22/1 -> Saturation Dynamic8/2
  Constant49/1 -> Saturation Dynamic7/1
  VVMC_MeterIndSpeedForCalcu_kph/1 -> [VVMC_MeterIndSpeedForCalcu_kph]
  VVMC_LongAcc_Gps/1 -> [VVMC_LongAcc_Gps]
  VTQD_DriverWhlTqDem_Nm/1 -> [VTQD_DriverWhlTqDem_Nm]
  VVMC_MSAActive_flg/1 -> [VVMC_MSAActive_flg]
  VINP_VehSpeed_kph/1 -> [VINP_VehSpeed_kph]
  VVMC_FeatSetSpdForCalcu_kph/1 -> [VVMC_FeatSetSpdForCalcu_kph]
  [VVMC_MSAWhlTqCal_Nm] -> VVMC_MSAWhlTqCal_Nm/1
  Constant19/1 -> Switch1/3
  Constant1/1 -> Switch1/2
  [VVMC_MSAReqAcc_mps2] -> Switch1/1
  [VVMC_FeatSetSpdForCalcu_kph] -> MVMC_MSATqDownTime_Y_s/1, MVMC_MSATqDownEndTq_Y_Nm/1
  AND5/1 -> Triggered Subsystem1/Trigger
  Cast To Single4/1 -> Switch5/3
  NOT4/1 -> OR/1
  Constant5/1 -> AND7/2
  [VTQD_LowIdleAccPedal_flg] -> AND7/3
  [VVMC_MSAInCtrlSpd_flg] -> AND8/2
  AND8/1 -> Detect Increase1/1
  Switch4/1 -> Switch10/3
  Add2/1 -> Switch/1, Switch6/1, Switch12/1, Relational Operator10/1, Switch4/1
  Relational Operator10/1 -> AND8/1
  [VVMC_MSATqDownEndTq_Nm] -> Divide4/1
  Detect Increase1/1 -> Switch4/2
  Divide4/1 -> Relational Operator10/2
  Constant9/1 -> Divide4/2
  [VVMC_MSAActive_flg] -> NOT4/1
  Constant6/1 -> Switch3/1
  OR/1 -> Switch3/2
  [VVMC_MSAPedalOvrd_flg] -> OR/2
  Switch5/1 -> Switch3/3
  AND7/1 -> Switch5/2
  Constant10/1 -> Switch5/1
  VVMC_TotalAvailBrkRgnTq_Nm/1 -> [VVMC_TotalAvailBrkRgnTq_Nm]
  [VVMC_TotalAvailBrkRgnTq_Nm] -> Max/2
  Max/1 -> Saturation Dynamic7/3
  [VVMC_MSAActive_flg] -> Detect Increase3/1
  Detect Increase3/1 -> Switch6/2
  [VVMC_LastMSAWhlTqCalW_Nm] -> Switch6/3
  [VVMC_FeatSetSpdForCalcu_kph] -> 1-D Lookup Table4/1
  [VVMC_MeterIndSpeedForCalcu_kph] -> Relational Operator8/1
  [VVMC_FeatSetSpdForCalcu_kph] -> Product13/1
  Constant2/1 -> Add6/1
  1-D Lookup Table4/1 -> Add6/2
  Add6/1 -> Product14/1
  Constant3/1 -> Product14/2
  Product14/1 -> Product13/2
  Product13/1 -> Relational Operator8/2
  Relational Operator8/1 -> [VVMC_MSAInCtrlSpd_flg]
  [VVMC_MSAInCtrlSpd_flg] -> NOT1/1
  [VVMC_MSAInCtrlSpd_flg] -> NOT2/1
  NOT2/1 -> AND7/1
  [VVMC_MSAPGainDeltaTq_Nm] -> Switch2/1
  Saturation Dynamic1/1 -> [VVMC_MSAWhlTqCal_Nm]  "VVMC_MSAWhlTqCal_Nm"
  Constant4/1 -> Switch2/2
  Constant7/1 -> Switch2/3
  Switch2/1 -> Add3/1
  Divide12/1 -> Switch7/3
  Constant65/1 -> Divide12/2
  Divide11/1 -> Add8/2
  Add8/1 -> Switch7/1
  Switch7/1 -> Add23/2
  Constant59/1 -> Add8/1
  Constant58/1 -> Divide11/1
  [VINP_VehSpeed_kph] -> Divide11/2, Switch7/2, Divide12/1
  Max1/1 -> Saturation Dynamic1/3
  [VVMC_TotalAvailBrkRgnTq_Nm] -> Max1/2
  Constant11/1 -> Saturation Dynamic1/1
  Constant8/1 -> Max1/1
  Add3/1 -> Saturation Dynamic1/2
  [VVMC_MSAPedalOvrd_flg] -> OR1/2
  OR1/1 -> Switch8/2
  Constant12/1 -> Switch8/1
  [VVMC_MSAActive_flg] -> NOT5/1
  NOT5/1 -> OR1/1
  MVMC_DISCDeltaTqPGain_Z_Nm/1 -> Switch8/3
